simulink model "MPC"  (R2024b)
settings: Solver=ode4  StartTime=0.0  StopTime=tsim  FixedStep=baseRate  RelTol=1e-6  AbsTol=1e-6
values from neighbouring files (symbols this model uses):
  IBLACK = 0.1996    [unpackData.m]
  IRED = 0.1982    [unpackData.m]
  m = m + 5    (= 4)    [unpackData.m]
  M = diag([1/m; 1/m; 1/I])    [unpackData.m]
  mBLACK = 11.3620    (= 11.362)    [unpackData.m]
  mRED = 11.2970    (= 11.297)    [unpackData.m]
  N = 0    [unpackData.m]
  Q = blkdiag(0.0001*eye(2), 0.00001)    [unpackData.m]
  R = diag([6;6;6])    [unpackData.m]
undefined symbols (not defined in the file or in its folder): a1, a2, a3, alpha, alpha_m, alpha_t, alphas, alphas_t, alphat, Am, b, b0, b1, b2, b3, baseRate, Bm, C, c, c1, c1t, c2, c2t, camera_FOV, camera_offset, Cm, d, dataRate, DiscIntNeverNeededParam, Dm, docking_face, docking_offset, drop_states_ARM, drop_states_BLACK, drop_states_BLUE, drop_states_RED, epsilon, epsilont, eta, F_black_X_nominal, F_black_Y_nominal, F_blue_X_nominal, F_blue_Y_nominal, F_max, F_red_X_nominal, F_red_Y_nominal, f_t, F_t, F_thrusters_BLACK, F_thrusters_BLUE, F_thrusters_RED, F_u, f_u, F_v, gamma, Gamma1_el, Gamma1_sh, Gamma1_wr, Gamma2_el, Gamma2_sh ... (+118)
libraries: simulink x33, nvidiaSharedBlocks x13, slpidlib x6, MainLibrary x5, dspsigops x3, dspinverses x3, nvidiaIMUSensorslib x1
(part 2 of 11)

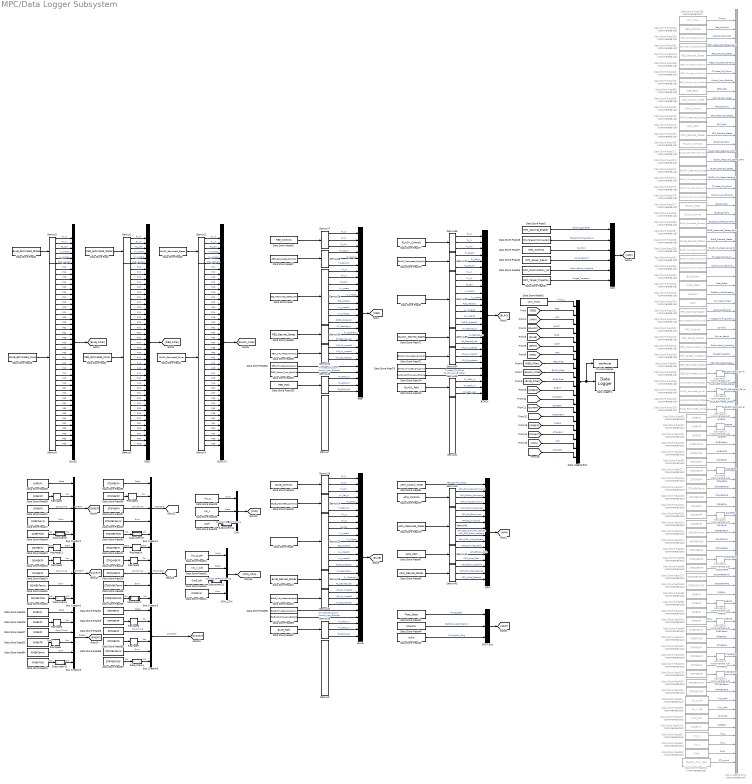
== system MPC/Data Logger Subsystem ==
  ARM : BusCreator  Inputs=16
  BLACK : BusCreator  Inputs=26
  BLACK2 : BusCreator  Inputs=42
  BLUE : BusCreator  Inputs=26
  BLUE2 : BusCreator  Inputs=42
  Bus Creator{1..4} (4 alike) : BusCreator  Inputs=5
  Bus Creator5 : BusCreator  Inputs=6
  Bus Creator6 : BusCreator  Inputs=6
  CNN : BusCreator  Inputs=3
  CNN_ZOH : BusCreator  Inputs=4
  Data Logger1 : MainLibrary/Data Logger  SystemSampleTime=-1  VariantActivationTime=update diagram  AllowFlexibleInterface=on  Latency=0  AutoFrameSizeCalculation=off
      settings: SourceProductName=SPOT Custom Library
  Data Logging Bus : BusCreator  Inputs=18
  Data Logging Bus1 : BusCreator  Commented=on  Inputs=85
  Data Store Read : DataStoreRead  DataStoreName=RED_Estimated_States  IndexOptions=Index vector (dialog)  Indices=1  OutputSizes=1
  Data Store Read1 : DataStoreRead  DataStoreName=MPC_Docking_Enabler  IndexOptions=Index vector (dialog)  Indices=1  OutputSizes=1
  Data Store Read10 : DataStoreRead  DataStoreName=STDQMEKFx  IndexOptions=Index vector (dialog)  Indices=1  OutputSizes=1
  Data Store Read100 : DataStoreRead  Commented=on  DataStoreName=Conf_zoh  IndexOptions=Index vector (dialog)  Indices=1  OutputSizes=1
  Data Store Read101 : DataStoreRead  Commented=on  DataStoreName=CNNError  IndexOptions=Index vector (dialog)  Indices=1  OutputSizes=1
  Data Store Read102 : DataStoreRead  Commented=on  DataStoreName=Float_State  IndexOptions=Index vector (dialog)  Indices=1  OutputSizes=1
  Data Store Read103 : DataStoreRead  Commented=on  DataStoreName=WhoAmI  IndexOptions=Index vector (dialog)  Indices=1  OutputSizes=1
  Data Store Read104 : DataStoreRead  Commented=on  DataStoreName=isSim  IndexOptions=Index vector (dialog)  Indices=1  OutputSizes=1
  Data Store Read105 : DataStoreRead  Commented=on  DataStoreName=RED_Estimated_Covar  IndexOptions=Index vector (dialog)  Indices=1  OutputSizes=1
  Data Store Read108 : DataStoreRead  Commented=on  DataStoreName=QMEKFerror  IndexOptions=Index vector (dialog)  Indices=1  OutputSizes=1
  Data Store Read11 : DataStoreRead  DataStoreName=QMEKFt  IndexOptions=Index vector (dialog)  Indices=1  OutputSizes=1
  Data Store Read114 : DataStoreRead  Commented=on  DataStoreName=DQMEKFerror  IndexOptions=Index vector (dialog)  Indices=1  OutputSizes=1
  Data Store Read115 : DataStoreRead  Commented=on  DataStoreName=DQMEKFNIS  IndexOptions=Index vector (dialog)  Indices=1  OutputSizes=1
  Data Store Read116 : DataStoreRead  Commented=on  DataStoreName=DQMEKFx  IndexOptions=Index vector (dialog)  Indices=1  OutputSizes=1
  Data Store Read117 : DataStoreRead  Commented=on  DataStoreName=STQMEKFP  IndexOptions=Index vector (dialog)  Indices=1  OutputSizes=1
  Data Store Read118 : DataStoreRead  Commented=on  DataStoreName=STQMEKFt  IndexOptions=Index vector (dialog)  Indices=1  OutputSizes=1
  Data Store Read119 : DataStoreRead  Commented=on  DataStoreName=QMEKFNIS  IndexOptions=Index vector (dialog)  Indices=1  OutputSizes=1
  Data Store Read12 : DataStoreRead  DataStoreName=DQMEKFx  IndexOptions=Index vector (dialog)  Indices=1  OutputSizes=1
  Data Store Read120 : DataStoreRead  Commented=on  DataStoreName=BLUE_Estimated_States  IndexOptions=Index vector (dialog)  Indices=1  OutputSizes=1
  Data Store Read122 : DataStoreRead  Commented=on  DataStoreName=MPC_Controls  IndexOptions=Index vector (dialog)  Indices=1  OutputSizes=1
  Data Store Read123 : DataStoreRead  Commented=on  DataStoreName=MPC_Solver_Result  IndexOptions=Index vector (dialog)  Indices=1  OutputSizes=1
  Data Store Read124 : DataStoreRead  Commented=on  DataStoreName=MPC_Target_Holding_Radius  IndexOptions=Index vector (dialog)  Indices=1  OutputSizes=1
  Data Store Read125 : DataStoreRead  Commented=on  DataStoreName=MPC_Optimization_Var  IndexOptions=Index vector (dialog)  Indices=1  OutputSizes=1
  Data Store Read126 : DataStoreRead  Commented=on  DataStoreName=BLUE_Estimated_Covar  IndexOptions=Index vector (dialog)  Indices=1  OutputSizes=1
  Data Store Read127 : DataStoreRead  Commented=on  DataStoreName=STQMEKFerror  IndexOptions=Index vector (dialog)  Indices=1  OutputSizes=1
  Data Store Read128 : DataStoreRead  Commented=on  DataStoreName=STQMEKFNIS  IndexOptions=Index vector (dialog)  Indices=1  OutputSizes=1
  Data Store Read129 : DataStoreRead  Commented=on  DataStoreName=DQMEKFP  IndexOptions=Index vector (dialog)  Indices=1  OutputSizes=1
  Data Store Read13 : DataStoreRead  DataStoreName=DQMEKFP  IndexOptions=Index vector (dialog)  Indices=1  OutputSizes=1
  Data Store Read130 : DataStoreRead  Commented=on  DataStoreName=QMEKFt  IndexOptions=Index vector (dialog)  Indices=1  OutputSizes=1
  Data Store Read131 : DataStoreRead  Commented=on  DataStoreName=DQMEKFt  IndexOptions=Index vector (dialog)  Indices=1  OutputSizes=1
  Data Store Read132 : DataStoreRead  Commented=on  DataStoreName=RMEKFt  IndexOptions=Index vector (dialog)  Indices=1  OutputSizes=1
  Data Store Read133 : DataStoreRead  DataStoreName=RED_Path  IndexOptions=Index vector (dialog)  Indices=1  OutputSizes=1
  Data Store Read134 : DataStoreRead  Commented=on  DataStoreName=RMEKFR  IndexOptions=Index vector (dialog)  Indices=1  OutputSizes=1
  Data Store Read135 : DataStoreRead  Commented=on  DataStoreName=BLACK_Estimated_Covar  IndexOptions=Index vector (dialog)  Indices=1  OutputSizes=1
  Data Store Read136 : DataStoreRead  Commented=on  DataStoreName=BLACK_Estimated_States  IndexOptions=Index vector (dialog)  Indices=1  OutputSizes=1
  Data Store Read137 : DataStoreRead  Commented=on  DataStoreName=STDQMEKFerror  IndexOptions=Index vector (dialog)  Indices=1  OutputSizes=1
  Data Store Read138 : DataStoreRead  Commented=on  DataStoreName=STDQMEKFNIS  IndexOptions=Index vector (dialog)  Indices=1  OutputSizes=1
  Data Store Read139 : DataStoreRead  Commented=on  DataStoreName=RED_Saturated_Controls  IndexOptions=Index vector (dialog)  Indices=1  OutputSizes=1
  Data Store Read14 : DataStoreRead  DataStoreName=DQMEKFt  IndexOptions=Index vector (dialog)  Indices=1  OutputSizes=1
  Data Store Read142 : DataStoreRead  Commented=on  DataStoreName=RMEKFNIS  IndexOptions=Index vector (dialog)  Indices=1  OutputSizes=1
  Data Store Read144 : DataStoreRead  Commented=on  DataStoreName=RED_Controls  IndexOptions=Index vector (dialog)  Indices=1  OutputSizes=1
  Data Store Read145 : DataStoreRead  Commented=on  DataStoreName=RED_Thruster_ON_Count  IndexOptions=Index vector (dialog)  Indices=1  OutputSizes=1
  Data Store Read146 : DataStoreRead  Commented=on  DataStoreName=RED_Control_Law_Enabler  IndexOptions=Index vector (dialog)  Indices=1  OutputSizes=1
  Data Store Read148 : DataStoreRead  Commented=on  DataStoreName=RED_Desired_States  IndexOptions=Index vector (dialog)  Indices=1  OutputSizes=1
  Data Store Read149 : DataStoreRead  Commented=on  DataStoreName=RED_IMU_Measurements  IndexOptions=Index vector (dialog)  Indices=1  OutputSizes=1
  Data Store Read15 : DataStoreRead  DataStoreName=RMEKFx  IndexOptions=Index vector (dialog)  Indices=1  OutputSizes=1
  Data Store Read150 : DataStoreRead  Commented=on  DataStoreName=MPC_Target_Trajectory  IndexOptions=Index vector (dialog)  Indices=1  OutputSizes=1
  Data Store Read151 : DataStoreRead  Commented=on  DataStoreName=MPC_Docking_Enabler  IndexOptions=Index vector (dialog)  Indices=1  OutputSizes=1
  Data Store Read152 : DataStoreRead  Commented=on  DataStoreName=STRMEKFx  IndexOptions=Index vector (dialog)  Indices=1  OutputSizes=1
  Data Store Read153 : DataStoreRead  Commented=on  DataStoreName=RED_Measured_States_RAW  IndexOptions=Index vector (dialog)  Indices=1  OutputSizes=1
  Data Store Read154 : DataStoreRead  Commented=on  DataStoreName=BLACK_CTL_Input  IndexOptions=Index vector (dialog)  Indices=1  OutputSizes=1
  Data Store Read155 : DataStoreRead  Commented=on  DataStoreName=BLUE_Controls  IndexOptions=Index vector (dialog)  Indices=1  OutputSizes=1
  Data Store Read156 : DataStoreRead  Commented=on  DataStoreName=BLUE_Saturated_Controls  IndexOptions=Index vector (dialog)  Indices=1  OutputSizes=1
  Data Store Read157 : DataStoreRead  Commented=on  DataStoreName=BLUE_Measured_States_RAW  IndexOptions=Index vector (dialog)  Indices=1  OutputSizes=1
  Data Store Read158 : DataStoreRead  Commented=on  DataStoreName=BLUE_Desired_States  IndexOptions=Index vector (dialog)  Indices=1  OutputSizes=1
  Data Store Read159 : DataStoreRead  Commented=on  DataStoreName=BLUE_IMU_Measurements  IndexOptions=Index vector (dialog)  Indices=1  OutputSizes=1
  Data Store Read16 : DataStoreRead  DataStoreName=RMEKFP  IndexOptions=Index vector (dialog)  Indices=1  OutputSizes=1
  Data Store Read160 : DataStoreRead  Commented=on  DataStoreName=BLUE_Thruster_ON_Count  IndexOptions=Index vector (dialog)  Indices=1  OutputSizes=1
  Data Store Read161 : DataStoreRead  Commented=on  DataStoreName=BLUE_Control_Law_Enabler  IndexOptions=Index vector (dialog)  Indices=1  OutputSizes=1
  Data Store Read162 : DataStoreRead  Commented=on  DataStoreName=ARM_Measured_States  IndexOptions=Index vector (dialog)  Indices=1  OutputSizes=1
  Data Store Read163 : DataStoreRead  Commented=on  DataStoreName=ARM_Controls  IndexOptions=Index vector (dialog)  Indices=1  OutputSizes=1
  Data Store Read164 : DataStoreRead  Commented=on  DataStoreName=BLUE_Path  IndexOptions=Index vector (dialog)  Indices=1  OutputSizes=1
  Data Store Read165 : DataStoreRead  Commented=on  DataStoreName=BLACK_Controls  IndexOptions=Index vector (dialog)  Indices=1  OutputSizes=1
  Data Store Read166 : DataStoreRead  Commented=on  DataStoreName=ARM_Control_Mode  IndexOptions=Index vector (dialog)  Indices=1  OutputSizes=1
  Data Store Read167 : DataStoreRead  Commented=on  DataStoreName=ARM_Desired_States  IndexOptions=Index vector (dialog)  Indices=1  OutputSizes=1
  Data Store Read168 : DataStoreRead  Commented=on  DataStoreName=STRMEKFP  IndexOptions=Index vector (dialog)  Indices=1  OutputSizes=1
  Data Store Read169 : DataStoreRead  Commented=on  DataStoreName=Univ_Time  IndexOptions=Index vector (dialog)  Indices=1  OutputSizes=1
  Data Store Read17 : DataStoreRead  DataStoreName=RMEKFt  IndexOptions=Index vector (dialog)  Indices=1  OutputSizes=1
  Data Store Read170 : DataStoreRead  Commented=on  DataStoreName=ARM_Path  IndexOptions=Index vector (dialog)  Indices=1  OutputSizes=1
  Data Store Read171 : DataStoreRead  Commented=on  DataStoreName=BLACK_Saturated_Controls  IndexOptions=Index vector (dialog)  Indices=1  OutputSizes=1
  Data Store Read172 : DataStoreRead  Commented=on  DataStoreName=BLACK_Measured_States_RAW  IndexOptions=Index vector (dialog)  Indices=1  OutputSizes=1
  Data Store Read173 : DataStoreRead  Commented=on  DataStoreName=BLACK_Desired_States  IndexOptions=Index vector (dialog)  Indices=1  OutputSizes=1
  Data Store Read174 : DataStoreRead  Commented=on  DataStoreName=BLACK_IMU_Measurements  IndexOptions=Index vector (dialog)  Indices=1  OutputSizes=1
  Data Store Read175 : DataStoreRead  Commented=on  DataStoreName=BLACK_Thruster_ON_Count  IndexOptions=Index vector (dialog)  Indices=1  OutputSizes=1
  Data Store Read176 : DataStoreRead  Commented=on  DataStoreName=BLACK_Control_Law_Enabler  IndexOptions=Index vector (dialog)  Indices=1  OutputSizes=1
  Data Store Read177 : DataStoreRead  Commented=on  DataStoreName=BLACK_Path  IndexOptions=Index vector (dialog)  Indices=1  OutputSizes=1
  Data Store Read178 : DataStoreRead  Commented=on  DataStoreName=STRMEKFt  IndexOptions=Index vector (dialog)  Indices=1  OutputSizes=1
  Data Store Read179 : DataStoreRead  Commented=on  DataStoreName=STRMEKFR  IndexOptions=Index vector (dialog)  Indices=1  OutputSizes=1
  Data Store Read18 : DataStoreRead  DataStoreName=STDQMEKFP  IndexOptions=Index vector (dialog)  Indices=1  OutputSizes=1
  Data Store Read180 : DataStoreRead  Commented=on  DataStoreName=STRMEKFerror  IndexOptions=Index vector (dialog)  Indices=1  OutputSizes=1
  Data Store Read181 : DataStoreRead  Commented=on  DataStoreName=STRMEKFNIS  IndexOptions=Index vector (dialog)  Indices=1  OutputSizes=1
  Data Store Read19 : DataStoreRead  DataStoreName=STDQMEKFt  IndexOptions=Index vector (dialog)  Indices=1  OutputSizes=1
  Data Store Read2 : DataStoreRead  DataStoreName=RED_Estimated_Covar  IndexOptions=Index vector (dialog)  Indices=1  OutputSizes=1
  Data Store Read20 : DataStoreRead  DataStoreName=RMEKFR  IndexOptions=Index vector (dialog)  Indices=1  OutputSizes=1
  Data Store Read21 : DataStoreRead  DataStoreName=RMEKFNIS  IndexOptions=Index vector (dialog)  Indices=1  OutputSizes=1
  Data Store Read22 : DataStoreRead  DataStoreName=STRMEKFx  IndexOptions=Index vector (dialog)  Indices=1  OutputSizes=1
  Data Store Read23 : DataStoreRead  DataStoreName=STRMEKFP  IndexOptions=Index vector (dialog)  Indices=1  OutputSizes=1
  Data Store Read24 : DataStoreRead  DataStoreName=BLUE_Desired_States  IndexOptions=Index vector (dialog)  Indices=1  OutputSizes=1
  Data Store Read25 : DataStoreRead  DataStoreName=BLUE_IMU_Measurements  IndexOptions=Index vector (dialog)  Indices=1  OutputSizes=1
  Data Store Read26 : DataStoreRead  DataStoreName=BLUE_Saturated_Controls  IndexOptions=Index vector (dialog)  Indices=1  OutputSizes=1
  Data Store Read27 : DataStoreRead  DataStoreName=MPC_Controls  IndexOptions=Index vector (dialog)  Indices=1  OutputSizes=1
  Data Store Read28 : DataStoreRead  DataStoreName=STRMEKFt  IndexOptions=Index vector (dialog)  Indices=1  OutputSizes=1
  Data Store Read29 : DataStoreRead  DataStoreName=Vis_q  IndexOptions=Index vector (dialog)  Indices=1  OutputSizes=1
  Data Store Read3 : DataStoreRead  DataStoreName=BLACK_Estimated_States  IndexOptions=Index vector (dialog)  Indices=1  OutputSizes=1
  Data Store Read30 : DataStoreRead  DataStoreName=Vis_x  IndexOptions=Index vector (dialog)  Indices=1  OutputSizes=1
  Data Store Read31 : DataStoreRead  DataStoreName=Vis_q_zoh  IndexOptions=Index vector (dialog)  Indices=1  OutputSizes=1
  Data Store Read32 : DataStoreRead  DataStoreName=Vis_x_zoh  IndexOptions=Index vector (dialog)  Indices=1  OutputSizes=1
  Data Store Read33 : DataStoreRead  DataStoreName=Conf  IndexOptions=Index vector (dialog)  Indices=1  OutputSizes=1
  Data Store Read34 : DataStoreRead  DataStoreName=Conf_zoh  IndexOptions=Index vector (dialog)  Indices=1  OutputSizes=1
  Data Store Read35 : DataStoreRead  DataStoreName=STQMEKFx  IndexOptions=Index vector (dialog)  Indices=1  OutputSizes=1
  Data Store Read36 : DataStoreRead  DataStoreName=STQMEKFP  IndexOptions=Index vector (dialog)  Indices=1  OutputSizes=1
  Data Store Read37 : DataStoreRead  DataStoreName=STQMEKFt  IndexOptions=Index vector (dialog)  Indices=1  OutputSizes=1
  Data Store Read38 : DataStoreRead  DataStoreName=QMEKFx  IndexOptions=Index vector (dialog)  Indices=1  OutputSizes=1
  Data Store Read39 : DataStoreRead  DataStoreName=QMEKFP  IndexOptions=Index vector (dialog)  Indices=1  OutputSizes=1
  Data Store Read4 : DataStoreRead  DataStoreName=BLACK_Estimated_Covar  IndexOptions=Index vector (dialog)  Indices=1  OutputSizes=1
  Data Store Read40 : DataStoreRead  DataStoreName=MPC_Solver_Result  IndexOptions=Index vector (dialog)  Indices=1  OutputSizes=1
  Data Store Read41 : DataStoreRead  DataStoreName=CNNError  IndexOptions=Index vector (dialog)  Indices=1  OutputSizes=1
  Data Store Read42 : DataStoreRead  DataStoreName=Float_State  IndexOptions=Index vector (dialog)  Indices=1  OutputSizes=1
  Data Store Read43 : DataStoreRead  DataStoreName=BLUE_Controls  IndexOptions=Index vector (dialog)  Indices=1  OutputSizes=1
  Data Store Read44 : DataStoreRead  DataStoreName=WhoAmI  IndexOptions=Index vector (dialog)  Indices=1  OutputSizes=1
  Data Store Read45 : DataStoreRead  DataStoreName=isSim  IndexOptions=Index vector (dialog)  Indices=1  OutputSizes=1
  Data Store Read46 : DataStoreRead  DataStoreName=MPC_Target_Holding_Radius  IndexOptions=Index vector (dialog)  Indices=1  OutputSizes=1
  Data Store Read47 : DataStoreRead  DataStoreName=QMEKFerror  IndexOptions=Index vector (dialog)  Indices=1  OutputSizes=1
  Data Store Read48 : DataStoreRead  DataStoreName=QMEKFNIS  IndexOptions=Index vector (dialog)  Indices=1  OutputSizes=1
  Data Store Read49 : DataStoreRead  DataStoreName=STQMEKFerror  IndexOptions=Index vector (dialog)  Indices=1  OutputSizes=1
  Data Store Read5 : DataStoreRead  DataStoreName=BLUE_Estimated_States  IndexOptions=Index vector (dialog)  Indices=1  OutputSizes=1
  Data Store Read50 : DataStoreRead  DataStoreName=STQMEKFNIS  IndexOptions=Index vector (dialog)  Indices=1  OutputSizes=1
  Data Store Read51 : DataStoreRead  DataStoreName=DQMEKFerror  IndexOptions=Index vector (dialog)  Indices=1  OutputSizes=1
  Data Store Read52 : DataStoreRead  DataStoreName=DQMEKFNIS  IndexOptions=Index vector (dialog)  Indices=1  OutputSizes=1
  Data Store Read53 : DataStoreRead  DataStoreName=MPC_Optimization_Var  IndexOptions=Index vector (dialog)  Indices=1  OutputSizes=1
  Data Store Read54 : DataStoreRead  DataStoreName=MPC_Target_Trajectory  IndexOptions=Index vector (dialog)  Indices=1  OutputSizes=1
  Data Store Read55 : DataStoreRead  DataStoreName=STDQMEKFerror  IndexOptions=Index vector (dialog)  Indices=1  OutputSizes=1
  Data Store Read56 : DataStoreRead  DataStoreName=STDQMEKFNIS  IndexOptions=Index vector (dialog)  Indices=1  OutputSizes=1
  Data Store Read57 : DataStoreRead  DataStoreName=RED_Saturated_Controls  IndexOptions=Index vector (dialog)  Indices=1  OutputSizes=1
  Data Store Read58 : DataStoreRead  DataStoreName=STRMEKFR  IndexOptions=Index vector (dialog)  Indices=1  OutputSizes=1
  Data Store Read59 : DataStoreRead  DataStoreName=STRMEKFerror  IndexOptions=Index vector (dialog)  Indices=1  OutputSizes=1
  Data Store Read6 : DataStoreRead  DataStoreName=BLUE_Estimated_Covar  IndexOptions=Index vector (dialog)  Indices=1  OutputSizes=1
  Data Store Read60 : DataStoreRead  DataStoreName=STRMEKFNIS  IndexOptions=Index vector (dialog)  Indices=1  OutputSizes=1
  Data Store Read61 : DataStoreRead  DataStoreName=RED_Controls  IndexOptions=Index vector (dialog)  Indices=1  OutputSizes=1
  Data Store Read62 : DataStoreRead  DataStoreName=RED_Thruster_ON_Count  IndexOptions=Index vector (dialog)  Indices=1  OutputSizes=1
  Data Store Read63 : DataStoreRead  DataStoreName=RED_Control_Law_Enabler  IndexOptions=Index vector (dialog)  Indices=1  OutputSizes=1
  Data Store Read64 : DataStoreRead  DataStoreName=RMEKFerror  IndexOptions=Index vector (dialog)  Indices=1  OutputSizes=1
  Data Store Read65 : DataStoreRead  DataStoreName=RED_Desired_States  IndexOptions=Index vector (dialog)  Indices=1  OutputSizes=1
  Data Store Read66 : DataStoreRead  DataStoreName=RED_IMU_Measurements  IndexOptions=Index vector (dialog)  Indices=1  OutputSizes=1
  Data Store Read67 : DataStoreRead  DataStoreName=BLUE_Path  IndexOptions=Index vector (dialog)  Indices=1  OutputSizes=1
  Data Store Read68 : DataStoreRead  DataStoreName=BLUE_Thruster_ON_Count  IndexOptions=Index vector (dialog)  Indices=1  OutputSizes=1
  Data Store Read69 : DataStoreRead  DataStoreName=BLUE_Control_Law_Enabler  IndexOptions=Index vector (dialog)  Indices=1  OutputSizes=1
  Data Store Read7 : DataStoreRead  DataStoreName=RED_Measured_States_RAW  IndexOptions=Index vector (dialog)  Indices=1  OutputSizes=1
  Data Store Read71 : DataStoreRead  DataStoreName=BLACK_Desired_States  IndexOptions=Index vector (dialog)  Indices=1  OutputSizes=1
  Data Store Read72 : DataStoreRead  DataStoreName=BLACK_IMU_Measurements  IndexOptions=Index vector (dialog)  Indices=1  OutputSizes=1
  Data Store Read73 : DataStoreRead  DataStoreName=BLACK_Thruster_ON_Count  IndexOptions=Index vector (dialog)  Indices=1  OutputSizes=1
  Data Store Read74 : DataStoreRead  DataStoreName=BLACK_Control_Law_Enabler  IndexOptions=Index vector (dialog)  Indices=1  OutputSizes=1
  Data Store Read75 : DataStoreRead  DataStoreName=BLACK_Saturated_Controls  IndexOptions=Index vector (dialog)  Indices=1  OutputSizes=1
  Data Store Read76 : DataStoreRead  DataStoreName=BLACK_Path  IndexOptions=Index vector (dialog)  Indices=1  OutputSizes=1
  Data Store Read77 : DataStoreRead  DataStoreName=BLACK_Controls  IndexOptions=Index vector (dialog)  Indices=1  OutputSizes=1
  Data Store Read78 : DataStoreRead  DataStoreName=ARM_Measured_States  IndexOptions=Index vector (dialog)  Indices=1  OutputSizes=1
  Data Store Read79 : DataStoreRead  DataStoreName=ARM_Controls  IndexOptions=Index vector (dialog)  Indices=1  OutputSizes=1
  Data Store Read8 : DataStoreRead  DataStoreName=BLACK_Measured_States_RAW  IndexOptions=Index vector (dialog)  Indices=1  OutputSizes=1
  Data Store Read80 : DataStoreRead  DataStoreName=ARM_Desired_States  IndexOptions=Index vector (dialog)  Indices=1  OutputSizes=1
  Data Store Read81 : DataStoreRead  DataStoreName=ARM_Control_Mode  IndexOptions=Index vector (dialog)  Indices=1  OutputSizes=1
  Data Store Read82 : DataStoreRead  Commented=on  DataStoreName=QMEKFx  IndexOptions=Index vector (dialog)  Indices=1  OutputSizes=1
  Data Store Read83 : DataStoreRead  Commented=on  DataStoreName=RED_Estimated_States  IndexOptions=Index vector (dialog)  Indices=1  OutputSizes=1
  Data Store Read84 : DataStoreRead  Commented=on  DataStoreName=STDQMEKFx  IndexOptions=Index vector (dialog)  Indices=1  OutputSizes=1
  Data Store Read85 : DataStoreRead  Commented=on  DataStoreName=STQMEKFx  IndexOptions=Index vector (dialog)  Indices=1  OutputSizes=1
  Data Store Read86 : DataStoreRead  Commented=on  DataStoreName=RMEKFerror  IndexOptions=Index vector (dialog)  Indices=1  OutputSizes=1
  Data Store Read87 : DataStoreRead  DataStoreName=ARM_Path  IndexOptions=Index vector (dialog)  Indices=1  OutputSizes=1
  Data Store Read88 : DataStoreRead  Commented=on  DataStoreName=RMEKFx  IndexOptions=Index vector (dialog)  Indices=1  OutputSizes=1
  Data Store Read89 : DataStoreRead  Commented=on  DataStoreName=RED_Path  IndexOptions=Index vector (dialog)  Indices=1  OutputSizes=1
  Data Store Read9 : DataStoreRead  DataStoreName=BLUE_Measured_States_RAW  IndexOptions=Index vector (dialog)  Indices=1  OutputSizes=1
  Data Store Read90 : DataStoreRead  Commented=on  DataStoreName=RMEKFP  IndexOptions=Index vector (dialog)  Indices=1  OutputSizes=1
  Data Store Read91 : DataStoreRead  DataStoreName=Univ_Time  IndexOptions=Index vector (dialog)  Indices=1  OutputSizes=1
  Data Store Read92 : DataStoreRead  Commented=on  DataStoreName=Vis_q  IndexOptions=Index vector (dialog)  Indices=1  OutputSizes=1
  Data Store Read93 : DataStoreRead  Commented=on  DataStoreName=Vis_x  IndexOptions=Index vector (dialog)  Indices=1  OutputSizes=1
  Data Store Read94 : DataStoreRead  Commented=on  DataStoreName=Vis_q_zoh  IndexOptions=Index vector (dialog)  Indices=1  OutputSizes=1
  Data Store Read95 : DataStoreRead  Commented=on  DataStoreName=STDQMEKFP  IndexOptions=Index vector (dialog)  Indices=1  OutputSizes=1
  Data Store Read96 : DataStoreRead  Commented=on  DataStoreName=STDQMEKFt  IndexOptions=Index vector (dialog)  Indices=1  OutputSizes=1
  Data Store Read97 : DataStoreRead  Commented=on  DataStoreName=QMEKFP  IndexOptions=Index vector (dialog)  Indices=1  OutputSizes=1
  Data Store Read98 : DataStoreRead  Commented=on  DataStoreName=Vis_x_zoh  IndexOptions=Index vector (dialog)  Indices=1  OutputSizes=1
  Data Store Read99 : DataStoreRead  Commented=on  DataStoreName=Conf  IndexOptions=Index vector (dialog)  Indices=1  OutputSizes=1
  Demux{1,3,5,41} (4 alike) : Demux  Outputs=6
  Demux2 : Demux  Outputs=36
  Demux{22..24,26..28,30..31,33..37,39..40,42..43,48} (18 alike) : Demux  Outputs=3
  Demux{7..9,25,29,38} (6 alike) : Demux  Outputs=9
  Demux4 : Demux  Outputs=36
  Demux6 : Demux  Outputs=36
  MPC : BusCreator  Inputs=6
  RED : BusCreator  Inputs=26
  RED2 : BusCreator  Inputs=42
  Reshape{1..8,13..14} (10 alike) : Reshape
  Reshape{9..12,17..23} (11 alike) : Reshape  Commented=on
  SPOT Bus : BusCreator  Inputs=3
  Subsystem1 : Subsystem
  Subsystem11 : Subsystem
  Subsystem13 : Subsystem
  Subsystem14 : Subsystem
  Subsystem17 : Subsystem
  Subsystem3 : Subsystem
  Subsystem4 : Subsystem
  Subsystem8 : Subsystem
  To Workspace1 : ToWorkspace  VariableName=dataPacket  SaveFormat=Timeseries  SampleTime=-1
      settings: Save2DSignal=2-D array (concatenate along first dimension)
  wires:
  Data Store Read24/1 -> Demux26/1
  Data Store Read43/1 -> Demux23/1
  Data Store Read26/1 -> Demux24/1
  Demux23/1 -> BLUE/1  "Fx_N"
  Demux23/2 -> BLUE/2  "Fy_N"
  Demux23/3 -> BLUE/3  "Tz_Nm"
  Demux24/1 -> BLUE/4  "Fx_Sat_N"
  Demux24/2 -> BLUE/5  "Fy_Sat_N"
  Demux24/3 -> BLUE/6  "Tz_Sat_Nm"
  Demux25/1 -> BLUE/7  "Px_m"
  Demux25/2 -> BLUE/8  "Py_m"
  Demux25/3 -> BLUE/9  "Rz_rad"
  Demux25/4 -> BLUE/10  "Vx_mpers"
  Demux25/5 -> BLUE/11  "Vy_mpers"
  Demux25/6 -> BLUE/12  "RzD_radpers"
  Demux25/7 -> BLUE/13  "Ax_mpers2"
  Demux25/8 -> BLUE/14  "Ay_mpers2"
  Demux25/9 -> BLUE/15  "RzDD_radpers2"
  Demux26/1 -> BLUE/16  "Px_Desired_m"
  Demux26/2 -> BLUE/17  "Py_Desired_m"
  Demux26/3 -> BLUE/18  "Rz_Desired_rad"
  Demux22/1 -> BLUE/19  "IMU_Ax_mpers2"
  Demux22/2 -> BLUE/20  "IMU_Ay_mpers2"
  Demux22/3 -> BLUE/21  "IMU_Gz_radpers"
  Data Store Read25/1 -> Demux22/1
  Data Store Read57/1 -> Demux28/1
  Data Store Read66/1 -> Demux31/1
  Data Store Read65/1 -> Demux30/1
  Data Store Read67/1 -> Demux33/1
  Data Store Read68/1 -> BLUE/22  "Thruster_ON_Count"
  Data Store Read69/1 -> BLUE/23  "Control_Law_Enabler"
  Data Store Read62/1 -> RED/22  "Thruster_ON_Count"
  Data Store Read63/1 -> RED/23  "Control_Law_Enabler"
  Demux29/9 -> RED/15  "RzDD_radpers2"
  Demux31/3 -> RED/21  "IMU_Gz_radpers"
  Demux28/3 -> RED/6  "Tz_Sat_Nm"
  Demux30/1 -> RED/16  "Px_Desired_m"
  Demux30/3 -> RED/18  "Rz_Desired_rad"
  Demux31/2 -> RED/20  "IMU_Ay_mpers2"
  Demux30/2 -> RED/17  "Py_Desired_m"
  Demux29/5 -> RED/11  "Vy_mpers"
  Demux29/4 -> RED/10  "Vx_mpers"
  Demux29/7 -> RED/13  "Ax_mpers2"
  Demux28/2 -> RED/5  "Fy_Sat_N"
  Demux29/6 -> RED/12  "RzD_radpers"
  Demux29/8 -> RED/14  "Ay_mpers2"
  Demux31/1 -> RED/19  "IMU_Ax_mpers2"
  Demux29/1 -> RED/7  "Px_m"
  Demux27/2 -> RED/2  "Fy_N"
  Demux29/2 -> RED/8  "Py_m"
  Demux27/1 -> RED/1  "Fx_N"
  Demux27/3 -> RED/3  "Tz_Nm"
  Demux28/1 -> RED/4  "Fx_Sat_N"
  Demux29/3 -> RED/9  "Rz_rad"
  Data Store Read61/1 -> Demux27/1
  Data Store Read72/1 -> Demux34/1
  Data Store Read75/1 -> Demux37/1
  Data Store Read76/1 -> Demux35/1
  Data Store Read77/1 -> Demux36/1
  Data Store Read71/1 -> Demux39/1
  Data Store Read73/1 -> BLACK/22  "Thruster_ON_Count"
  Data Store Read74/1 -> BLACK/23  "Control_Law_Enabler"
  Demux35/1 -> BLACK/24  "Px_Path_m"
  Demux35/2 -> BLACK/25  "Py_Path_m"
  Demux35/3 -> BLACK/26  "Rz_Path_rad"
  Demux34/3 -> BLACK/21  "IMU_Gz_radpers"
  Demux34/2 -> BLACK/20  "IMU_Ay_mpers2"
  Demux34/1 -> BLACK/19  "IMU_Ax_mpers2"
  Demux39/3 -> BLACK/18  "Rz_Desired_rad"
  Demux39/2 -> BLACK/17  "Py_Desired_m"
  Demux39/1 -> BLACK/16  "Px_Desired_m"
  Demux38/9 -> BLACK/15  "RzDD_radpers2"
  Demux38/8 -> BLACK/14  "Ay_mpers2"
  Demux38/7 -> BLACK/13  "Ax_mpers2"
  Demux38/6 -> BLACK/12  "RzD_radpers"
  Demux38/5 -> BLACK/11  "Vy_mpers"
  Demux38/4 -> BLACK/10  "Vx_mpers"
  Demux38/3 -> BLACK/9  "Rz_rad"
  Demux38/2 -> BLACK/8  "Py_m"
  Demux38/1 -> BLACK/7  "Px_m"
  Demux37/3 -> BLACK/6  "Tz_Sat_Nm"
  Demux37/2 -> BLACK/5  "Fy_Sat_N"
  Demux37/1 -> BLACK/4  "Fx_Sat_N"
  Demux36/3 -> BLACK/3  "Tz_Nm"
  Demux36/2 -> BLACK/2  "Fy_N"
  Demux36/1 -> BLACK/1  "Fx_N"
  Data Store Read87/1 -> Demux42/1
  Data Store Read79/1 -> Demux40/1
  Data Store Read78/1 -> Demux41/1
  Data Store Read80/1 -> Demux43/1
  Data Store Read81/1 -> ARM/1  "ARM_Control_Mode"
  Demux40/1 -> ARM/2  "ARM_Shoulder_Command"
  Demux40/2 -> ARM/3  "ARM_Elbow_Command"
  Demux40/3 -> ARM/4  "ARM_Wrist_Command"
  Demux41/1 -> ARM/5  "ARM_Rz_Shoulder_rad"
  Demux41/2 -> ARM/6  "ARM_Rz_Elbow_rad"
  Demux41/3 -> ARM/7  "ARM_Rz_Wrist_rad"
  Demux41/4 -> ARM/8  "ARM_RzD_Shoulder_radpers"
  Demux41/5 -> ARM/9  "ARM_RzD_Elbow_radpers"
  Demux41/6 -> ARM/10  "ARM_RzD_Wrist_radpers"
  Demux42/1 -> ARM/11  "ARM_Shoulder_Path"
  Demux42/2 -> ARM/12  "ARM_Elbow_Path"
  Demux42/3 -> ARM/13  "ARM_Wrist_Path"
  Demux43/1 -> ARM/14  "ARM_Elbow_Desired"
  Demux43/2 -> ARM/15  "ARM_Shoulder_Desired"
  Demux43/3 -> ARM/16  "ARM_Wrist_Desired"
  RED/1 -> [RED]
  ARM/1 -> [ARM]
  BLACK/1 -> [BLACK]
  BLUE/1 -> [BLUE]
  Demux48/1 -> RED/24  "Px_Path_m"
  Demux48/2 -> RED/25  "Py_Path_m"
  Demux48/3 -> RED/26  "Rz_Path_rad"
  Data Store Read133/1 -> Demux48/1
  Data Store Read42/1 -> SPOT Bus/1  "Float_State"
  SPOT Bus/1 -> [SPOT]
  Data Store Read45/1 -> SPOT Bus/3  "Simulation_Flag"
  Data Store Read44/1 -> SPOT Bus/2  "Platform_Identification"
  [MPC] -> Data Logging Bus/7  "MPC"
  [RED] -> Data Logging Bus/2  "RED"
  [SPOT] -> Data Logging Bus/6  "SPOT"
  [ARM] -> Data Logging Bus/3  "ARM"
  [BLUE] -> Data Logging Bus/5  "BLUE"
  [BLACK] -> Data Logging Bus/4  "BLACK"
  Data Store Read91/1 -> Data Logging Bus/1  "Time_s"
  MPC/1 -> [MPC]
  Data Store Read1/1 -> MPC/1  "Docking_Enabler"
  Data Store Read54/1 -> MPC/6  "Target_Trajectory"
  Data Store Read53/1 -> MPC/5  "Optimization_Variable"
  Data Store Read40/1 -> MPC/4  "Solver_Result"
  Data Store Read46/1 -> MPC/2  "Target_Holding_Radius"
  Data Store Read27/1 -> MPC/3  "Controls"
  Data Store Read/1 -> Demux1/1
  Data Store Read2/1 -> Demux2/1
  Demux1/6 -> RED2/6  "RzD_radpers"
  Demux1/5 -> RED2/5  "Vy_mpers"
  Demux1/4 -> RED2/4  "Vx_mpers"
  Demux1/3 -> RED2/3  "Rz_rad"
  Demux1/2 -> RED2/2  "Py_m"
  Demux1/1 -> RED2/1  "Px_m"
  Demux2/1 -> RED2/7  "P11"
  Demux2/2 -> RED2/8  "P12"
  Demux2/3 -> RED2/9  "P13"
  Demux2/4 -> RED2/10  "P14"
  Demux2/5 -> RED2/11  "P15"
  Demux2/6 -> RED2/12  "P16"
  Demux2/7 -> RED2/13  "P21"
  Demux2/8 -> RED2/14  "P22"
  Demux2/9 -> RED2/15  "P23"
  Demux2/10 -> RED2/16  "P24"
  Demux2/11 -> RED2/17  "P25"
  Demux2/12 -> RED2/18  "P26"
  Demux2/13 -> RED2/19  "P31"
  Demux2/14 -> RED2/20  "P32"
  Demux2/15 -> RED2/21  "P33"
  Demux2/16 -> RED2/22  "P34"
  Demux2/17 -> RED2/23  "P35"
  Demux2/18 -> RED2/24  "P36"
  Demux2/19 -> RED2/25  "P41"
  Demux2/20 -> RED2/26  "P42"
  Demux2/21 -> RED2/27  "P43"
  Demux2/22 -> RED2/28  "P44"
  Demux2/23 -> RED2/29  "P45"
  Demux2/24 -> RED2/30  "P46"
  Demux2/25 -> RED2/31  "P51"
  Demux2/26 -> RED2/32  "P52"
  Demux2/27 -> RED2/33  "P53"
  Demux2/28 -> RED2/34  "P54"
  Demux2/29 -> RED2/35  "P55"
  Demux2/30 -> RED2/36  "P56"
  Demux2/31 -> RED2/37  "P61"
  Demux2/32 -> RED2/38  "P62"
  Demux2/33 -> RED2/39  "P63"
  Demux2/34 -> RED2/40  "P64"
  Demux2/35 -> RED2/41  "P65"
  Demux2/36 -> RED2/42  "P66"
  RED2/1 -> [RED_Filter]
  Demux4/13 -> BLACK2/19  "P31"
  Demux4/27 -> BLACK2/33  "P53"
  Demux4/18 -> BLACK2/24  "P36"
  Demux4/26 -> BLACK2/32  "P52"
  Demux3/6 -> BLACK2/6  "RzD_radpers"
  Demux3/5 -> BLACK2/5  "Vy_mpers"
  Demux4/2 -> BLACK2/8  "P12"
  Demux4/14 -> BLACK2/20  "P32"
  Demux4/24 -> BLACK2/30  "P46"
  Demux4/16 -> BLACK2/22  "P34"
  Demux3/2 -> BLACK2/2  "Py_m"
  Demux4/29 -> BLACK2/35  "P55"
  Demux4/31 -> BLACK2/37  "P61"
  Demux4/10 -> BLACK2/16  "P24"
  Demux3/4 -> BLACK2/4  "Vx_mpers"
  Demux4/9 -> BLACK2/15  "P23"
  Demux3/3 -> BLACK2/3  "Rz_rad"
  Demux4/12 -> BLACK2/18  "P26"
  Demux4/22 -> BLACK2/28  "P44"
  Data Store Read3/1 -> Demux3/1
  Demux4/23 -> BLACK2/29  "P45"
  Demux4/3 -> BLACK2/9  "P13"
  Demux4/21 -> BLACK2/27  "P43"
  Demux4/30 -> BLACK2/36  "P56"
  Demux4/5 -> BLACK2/11  "P15"
  Demux4/17 -> BLACK2/23  "P35"
  Demux4/20 -> BLACK2/26  "P42"
  Demux4/6 -> BLACK2/12  "P16"
  Demux4/19 -> BLACK2/25  "P41"
  Data Store Read4/1 -> Demux4/1
  Demux4/4 -> BLACK2/10  "P14"
  Demux4/7 -> BLACK2/13  "P21"
  BLACK2/1 -> [BLACK_Filter]
  Demux4/25 -> BLACK2/31  "P51"
  Demux4/28 -> BLACK2/34  "P54"
  Demux4/8 -> BLACK2/14  "P22"
  Demux4/15 -> BLACK2/21  "P33"
  Demux4/11 -> BLACK2/17  "P25"
  Demux3/1 -> BLACK2/1  "Px_m"
  Demux4/1 -> BLACK2/7  "P11"
  Demux5/1 -> BLUE2/1  "Px_m"
  Demux6/25 -> BLUE2/31  "P51"
  BLUE2/1 -> [BLUE_Filter]
  Data Store Read6/1 -> Demux6/1
  Demux6/4 -> BLUE2/10  "P14"
  Demux6/19 -> BLUE2/25  "P41"
  Demux6/28 -> BLUE2/34  "P54"
  Demux6/30 -> BLUE2/36  "P56"
  Demux6/6 -> BLUE2/12  "P16"
  Demux6/21 -> BLUE2/27  "P43"
  Demux6/5 -> BLUE2/11  "P15"
  Demux6/22 -> BLUE2/28  "P44"
  Demux5/3 -> BLUE2/3  "Rz_rad"
  Demux6/12 -> BLUE2/18  "P26"
  Demux6/8 -> BLUE2/14  "P22"
  Demux5/2 -> BLUE2/2  "Py_m"
  Demux6/1 -> BLUE2/7  "P11"
  Demux6/16 -> BLUE2/22  "P34"
  Demux6/31 -> BLUE2/37  "P61"
  Demux6/10 -> BLUE2/16  "P24"
  Demux6/3 -> BLUE2/9  "P13"
  Demux6/9 -> BLUE2/15  "P23"
  Demux5/4 -> BLUE2/4  "Vx_mpers"
  Demux5/6 -> BLUE2/6  "RzD_radpers"
  Demux6/20 -> BLUE2/26  "P42"
  Demux6/24 -> BLUE2/30  "P46"
  Demux6/7 -> BLUE2/13  "P21"
  Demux6/11 -> BLUE2/17  "P25"
  Demux6/18 -> BLUE2/24  "P36"
  Demux6/29 -> BLUE2/35  "P55"
  Demux6/27 -> BLUE2/33  "P53"
  Demux6/23 -> BLUE2/29  "P45"
  Demux6/13 -> BLUE2/19  "P31"
  Demux6/15 -> BLUE2/21  "P33"
  Demux6/26 -> BLUE2/32  "P52"
  Demux6/2 -> BLUE2/8  "P12"
  Demux5/5 -> BLUE2/5  "Vy_mpers"
  Data Store Read5/1 -> Demux5/1
  Demux6/17 -> BLUE2/23  "P35"
  Demux6/14 -> BLUE2/20  "P32"
  Demux4/32 -> BLACK2/38  "P62"
  Demux4/33 -> BLACK2/39  "P63"
  Demux4/34 -> BLACK2/40  "P64"
  Demux4/35 -> BLACK2/41  "P65"
  Demux4/36 -> BLACK2/42  "P66"
  Demux6/32 -> BLUE2/38  "P62"
  Demux6/33 -> BLUE2/39  "P63"
  Demux6/34 -> BLUE2/40  "P64"
  Demux6/35 -> BLUE2/41  "P65"
  Demux6/36 -> BLUE2/42  "P66"
  [RED_Filter] -> Data Logging Bus/8  "RED_Filter"
  [BLACK_Filter] -> Data Logging Bus/9  "BLACK_Filter"
  [BLUE_Filter] -> Data Logging Bus/10  "BLUE_Filter"
  Demux33/1 -> BLUE/24  "Px_Path_m"
  Demux33/2 -> BLUE/25  "Py_Path_m"
  Demux33/3 -> BLUE/26  "Rz_Path_rad"
  Data Store Read8/1 -> Demux38/1
  Data Store Read7/1 -> Demux29/1
  Data Store Read9/1 -> Demux25/1
  Bus Creator3/1 -> [STDQMEKF]  "STDQMEKF"
  Bus Creator4/1 -> [STQMEKF]  "STQMEKF"
  Data Store Read39/1 -> Reshape1/1
  Reshape1/1 -> Bus Creator1/2  "Cov"
  CNN/1 -> [CNN]
  Bus Creator1/1 -> [QMEKF]  "QMEKF"
  Bus Creator2/1 -> [DQMEKF]  "DQMEKF"
  Data Store Read33/1 -> Subsystem14/1(In1)  "Confidence"
  Bus Creator6/1 -> [STRMEKF]  "STRMEKF"
  Bus Creator5/1 -> [RMEKF]  "RMEKF"
  Data Store Read11/1 -> Bus Creator1/3  "CompTime"
  Data Store Read38/1 -> Bus Creator1/1  "State"
  [QMEKF] -> Data Logging Bus/11  "QMEKF"
  [STQMEKF] -> Data Logging Bus/12  "STQMEKF"
  [DQMEKF] -> Data Logging Bus/13  "DQMEKF"
  [STDQMEKF] -> Data Logging Bus/14  "STDQMEKF"
  [RMEKF] -> Data Logging Bus/15  "RMEKF"
  [STRMEKF] -> Data Logging Bus/16  "STRMEKF"
  [CNN] -> Data Logging Bus/17  "CNN"
  Data Store Read32/1 -> CNN_ZOH/2  "State"
  CNN_ZOH/1 -> [CNN_ZOH]
  Data Store Read31/1 -> CNN_ZOH/1  "Quat"
  Data Store Read34/1 -> Subsystem13/1(In1)  "Confidence"
  [CNN_ZOH] -> Data Logging Bus/18  "CNN_ZOH"
  Data Store Read41/1 -> CNN_ZOH/4  "Error"
  Data Store Read47/1 -> Bus Creator1/4  "Error"
  Data Store Read48/1 -> Subsystem8/1(In1)  "NIS"
  Data Store Read35/1 -> Bus Creator4/1  "State"
  Data Store Read36/1 -> Reshape4/1
  Data Store Read37/1 -> Bus Creator4/3  "CompTime"
  Data Store Read49/1 -> Bus Creator4/4  "Error"
  Data Store Read50/1 -> Subsystem17/1(In1)  "NIS"
  Reshape4/1 -> Bus Creator4/2  "Cov"
  Reshape2/1 -> Bus Creator2/2  "Cov"
  Data Store Read52/1 -> Subsystem3/1(In1)  "NIS"
  Data Store Read12/1 -> Reshape13/1  "State"
  Data Store Read14/1 -> Bus Creator2/3  "CompTime"
  Data Store Read51/1 -> Bus Creator2/4  "Error"
  Data Store Read13/1 -> Reshape2/1
  Reshape3/1 -> Bus Creator3/2  "Cov"
  Data Store Read56/1 -> Subsystem1/1(In1)  "NIS"
  Data Store Read10/1 -> Reshape14/1  "State"
  Data Store Read19/1 -> Bus Creator3/3  "CompTime"
  Data Store Read55/1 -> Bus Creator3/4  "Error"
  Data Store Read18/1 -> Reshape3/1
  Reshape5/1 -> Bus Creator5/2  "Cov"
  Data Store Read21/1 -> Subsystem11/1(In1)  "NIS"
  Data Store Read15/1 -> Bus Creator5/1  "State"
  Data Store Read17/1 -> Bus Creator5/3  "CompTime"
  Data Store Read64/1 -> Bus Creator5/5  "Error"
  Reshape6/1 -> Bus Creator6/2  "Cov"
  Data Store Read60/1 -> Subsystem4/1(In1)  "NIS"
  Data Store Read22/1 -> Bus Creator6/1  "State"
  Data Store Read28/1 -> Bus Creator6/3  "CompTime"
  Data Store Read59/1 -> Bus Creator6/5  "Error"
  Data Store Read16/1 -> Reshape5/1
  Data Store Read23/1 -> Reshape6/1
  Data Store Read58/1 -> Reshape7/1
  Reshape7/1 -> Bus Creator6/4  "Rot"
  Data Store Read20/1 -> Reshape8/1  "Error"
  Reshape8/1 -> Bus Creator5/4  "Rot"
  Data Store Read154/1 -> Data Logging Bus1/85  "CTL_Input"
  Data Store Read169/1 -> Data Logging Bus1/1  "Time_s"
  Data Store Read144/1 -> Data Logging Bus1/2  "Red_Controls"
  Data Store Read139/1 -> Data Logging Bus1/3  "Red_Controls_Sat"
  Data Store Read153/1 -> Data Logging Bus1/4  "RED_Measured_States_RAW"
  Data Store Read148/1 -> Data Logging Bus1/5  "RED_Desired_States"
  Data Store Read149/1 -> Data Logging Bus1/6  "RED_IMU_Measurements"
  Data Store Read145/1 -> Data Logging Bus1/7  "Thruster_ON_Count"
  Data Store Read146/1 -> Data Logging Bus1/8  "Control_Law_Enabler"
  Data Store Read89/1 -> Data Logging Bus1/9  "RED_Path"
  Data Store Read166/1 -> Data Logging Bus1/10  "ARM_Control_Mode"
  Data Store Read163/1 -> Data Logging Bus1/11  "ARM_Controls"
  Data Store Read162/1 -> Data Logging Bus1/12  "ARM_Measured_States"
  Data Store Read170/1 -> Data Logging Bus1/13  "ARM_Path"
  Data Store Read167/1 -> Data Logging Bus1/14  "ARM_Desired_States"
  Data Store Read165/1 -> Data Logging Bus1/15  "BLACK_Controls"
  Data Store Read171/1 -> Data Logging Bus1/16  "BLACK_Saturated_Controls"
  Data Store Read172/1 -> Data Logging Bus1/17  "BLACK_Measured_States_RAW"
  Data Store Read173/1 -> Data Logging Bus1/18  "BLACK_Desired_States"
  Data Store Read174/1 -> Data Logging Bus1/19  "BLACK_IMU_Measurements"
  Data Store Read175/1 -> Data Logging Bus1/20  "Thruster_ON_Count"
  Data Store Read176/1 -> Data Logging Bus1/21  "Control_Law_Enabler"
  Data Store Read177/1 -> Data Logging Bus1/22  "BLACK_Path"
  Data Store Read155/1 -> Data Logging Bus1/23  "BLUE_Controls"
  Data Store Read156/1 -> Data Logging Bus1/24  "BLUE_Saturated_Controls"
  Data Store Read157/1 -> Data Logging Bus1/25  "BLUE_Measured_States_RAW"
  Data Store Read158/1 -> Data Logging Bus1/26  "BLUE_Desired_States"
  Data Store Read159/1 -> Data Logging Bus1/27  "BLUE_IMU_Measurements"
  Data Store Read160/1 -> Data Logging Bus1/28  "Thruster_ON_Count"
  Data Store Read161/1 -> Data Logging Bus1/29  "Control_Law_Enabler"
  Data Store Read164/1 -> Data Logging Bus1/30
  Data Store Read102/1 -> Data Logging Bus1/31  "Float_State"
  Data Store Read103/1 -> Data Logging Bus1/32  "Platform_Identification"
  Data Store Read104/1 -> Data Logging Bus1/33  "Simulation_Flag"
  Data Store Read124/1 -> Data Logging Bus1/35  "Target_Holding_Radius"
  Data Store Read150/1 -> Data Logging Bus1/39  "Target_Trajectory"
  Data Store Read122/1 -> Data Logging Bus1/36  "Controls"
  Data Store Read123/1 -> Data Logging Bus1/37  "Solver_Result"
  Data Store Read151/1 -> Data Logging Bus1/34  "Docking_Enabler"
  Data Store Read125/1 -> Data Logging Bus1/38  "Optimization_Variable"
  Data Store Read83/1 -> Data Logging Bus1/40  "RED_Estimated_States"
  Data Store Read105/1 -> Reshape17/1
  Reshape17/1 -> Data Logging Bus1/41  "RED_Estimated_Covar"
  Data Store Read120/1 -> Data Logging Bus1/44  "BLUE_Estimated_States"
  Data Store Read126/1 -> Reshape19/1
  Data Store Read135/1 -> Reshape18/1
  Data Store Read136/1 -> Data Logging Bus1/42  "BLACK_Estimated_States"
  Reshape18/1 -> Data Logging Bus1/43  "BLACK_Estimated_Covar"
  Reshape19/1 -> Data Logging Bus1/45  "BLUE_Estimated_Covar"
  Data Store Read82/1 -> Data Logging Bus1/46  "QMEKFx"
  Data Store Read97/1 -> Reshape20/1
  Reshape20/1 -> Data Logging Bus1/47  "QMEKFP"
  Data Store Read130/1 -> Data Logging Bus1/48  "QMEKFt"
  Data Store Read108/1 -> Data Logging Bus1/49  "QMEKFerror"
  Data Store Read119/1 -> Data Logging Bus1/50  "QMEKFNIS"
  Data Store Read128/1 -> Data Logging Bus1/55  "STQMEKFNIS"
  Data Store Read127/1 -> Data Logging Bus1/54  "STQMEKFerror"
  Data Store Read117/1 -> Reshape9/1
  Data Store Read118/1 -> Data Logging Bus1/53  "STQMEKFt"
  Reshape9/1 -> Data Logging Bus1/52  "STQMEKFP"
  Data Store Read85/1 -> Data Logging Bus1/51  "STQMEKFx"
  Reshape12/1 -> Data Logging Bus1/57  "DQMEKFP"
  Data Store Read116/1 -> Data Logging Bus1/56  "DQMEKFx"
  Data Store Read131/1 -> Data Logging Bus1/58  "DQMEKFt"
  Data Store Read114/1 -> Data Logging Bus1/59  "DQMEKFerror"
  Data Store Read115/1 -> Data Logging Bus1/60  "DQMEKFNIS"
  Data Store Read129/1 -> Reshape12/1
  Data Store Read137/1 -> Data Logging Bus1/64  "STDQMEKFerror"
  Data Store Read95/1 -> Reshape11/1
  Data Store Read138/1 -> Data Logging Bus1/65  "STDQMEKFNIS"
  Data Store Read96/1 -> Data Logging Bus1/63  "STDQMEKFt"
  Data Store Read84/1 -> Data Logging Bus1/61  "STDQMEKFx"
  Reshape11/1 -> Data Logging Bus1/62  "STDQMEKFP"
  Data Store Read134/1 -> Reshape21/1  "Error"
  Data Store Read142/1 -> Data Logging Bus1/71  "RMEKFNIS"
  Data Store Read132/1 -> Data Logging Bus1/68  "RMEKFt"
  Data Store Read86/1 -> Data Logging Bus1/70  "RMEKFerror"
  Data Store Read90/1 -> Reshape10/1
  Data Store Read88/1 -> Data Logging Bus1/66  "RMEKFx"
  Data Store Read178/1 -> Data Logging Bus1/74  "STRMEKFt"
  Data Store Read181/1 -> Data Logging Bus1/77  "STRMEKFNIS"
  Data Store Read168/1 -> Reshape22/1
  Data Store Read180/1 -> Data Logging Bus1/76  "STRMEKFerror"
  Data Store Read179/1 -> Reshape23/1
  Reshape22/1 -> Data Logging Bus1/73  "STRMEKFP"
  Reshape23/1 -> Data Logging Bus1/75  "STRMEKFR"
  Data Store Read152/1 -> Data Logging Bus1/72  "STRMEKFx"
  Reshape10/1 -> Data Logging Bus1/67  "RMEKFP"
  Reshape21/1 -> Data Logging Bus1/69  "RMEKFR"
  Data Store Read92/1 -> Data Logging Bus1/82  "Vis_q"
  Data Store Read94/1 -> Data Logging Bus1/78  "Vis_q_zoh"
  Data Store Read93/1 -> Data Logging Bus1/83  "Vis_x"
  Data Store Read98/1 -> Data Logging Bus1/79  "Vis_x_zoh"
  Data Store Read101/1 -> Data Logging Bus1/81  "CNNError"
  Data Store Read100/1 -> Data Logging Bus1/80  "Conf_zoh"
  Data Store Read99/1 -> Data Logging Bus1/84  "Conf"
  Data Logging Bus/1 -> To Workspace1/1, Data Logger1/1
  Subsystem8/1(y) -> Bus Creator1/5  "NIS"
  Subsystem3/1(y) -> Bus Creator2/5  "NIS"
  Subsystem11/1(y) -> Bus Creator5/6  "NIS"
  Subsystem4/1(y) -> Bus Creator6/6  "NIS"
  Subsystem1/1(y) -> Bus Creator3/5  "NIS"
  Subsystem17/1(y) -> Bus Creator4/5  "NIS"
  Subsystem13/1(y) -> CNN_ZOH/3  "Confidence"
  Subsystem14/1(y) -> CNN/3  "Confidence"
  Data Store Read30/1 -> CNN/2  "State"
  Data Store Read29/1 -> CNN/1  "Quat"
  Reshape13/1 -> Bus Creator2/1  "State"
  Reshape14/1 -> Bus Creator3/1  "State"

== system MPC/Debugger1 ==
  Change BLACK Behavior : Subsystem  TreatAsAtomicUnit=on
  Change BLUE Behavior : Subsystem  TreatAsAtomicUnit=on
  Change RED Behavior : Subsystem  TreatAsAtomicUnit=on
  Data Store Read : DataStoreRead  DataStoreName=WhoAmI  IndexOptions=Index vector (dialog)  Indices=1  OutputSizes=1
  Data Store Read1 : DataStoreRead  DataStoreName=isSim  IndexOptions=Index vector (dialog)  Indices=1  OutputSizes=1
  This IF block determines whether or not to run the BLACK sim/exp : If  NumInputs=2  IfExpression=u1 == 2 & u2 == 0  ShowElse=off
  This IF block determines whether or not to run the BLUE sim/exp : If  NumInputs=2  IfExpression=u1 == 3 & u2 == 0  ShowElse=off
  "This IF block determines whether or not to run the RED sim/exp " : If  NumInputs=2  IfExpression=u1 == 1 & u2 == 0  ShowElse=off
  wires:
  Data Store Read1/1 -> This IF block determines whether or not to run the BLACK sim/exp/2, This IF block determines whether or not to run the BLUE sim/exp/2, "This IF block determines whether or not to run the RED sim/exp "/2
  Data Store Read/1 -> This IF block determines whether or not to run the BLUE sim/exp/1, This IF block determines whether or not to run the BLACK sim/exp/1, "This IF block determines whether or not to run the RED sim/exp "/1
  "This IF block determines whether or not to run the RED sim/exp "/1 -> Change RED Behavior/Action
  This IF block determines whether or not to run the BLACK sim/exp/1 -> Change BLACK Behavior/Action
  This IF block determines whether or not to run the BLUE sim/exp/1 -> Change BLUE Behavior/Action

== system MPC/Float Code ==
  note: In this subsection, the "if" statements are used to determine two things: 1) whether or not a simulation is begin performed,
      | then 2) if an experiment is being performed, then which platform is the diagram compiled on. The "IdentifyPlatform" variable
      | is obtained from a text file location on each platform; each text file contains a unique identifier for each platform.
  Data Store Read : DataStoreRead  DataStoreName=isSim  IndexOptions=Index vector (dialog)  Indices=1  OutputSizes=1
  Enable Pucks : Subsystem  TreatAsAtomicUnit=on
  This IF block determines whether or not to run the exp code : If  IfExpression=u1 == 0  ShowElse=off
  wires:
  Data Store Read/1 -> This IF block determines whether or not to run the exp code/1
  This IF block determines whether or not to run the exp code/1 -> Enable Pucks/Action

== system MPC/Gyro.//Accel. Code ==
  Data Store Read1 : DataStoreRead  DataStoreName=isSim  IndexOptions=Index vector (dialog)  Indices=1  OutputSizes=1
  Log Gyro/Accel : Subsystem  TreatAsAtomicUnit=on
  This IF block determines whether or not to run the exp code : If  IfExpression=u1 == 0  ShowElse=off
  wires:
  This IF block determines whether or not to run the exp code/1 -> Log Gyro/Accel/Action
  Data Store Read1/1 -> This IF block determines whether or not to run the exp code/1

== system MPC/Manipulator Encoder Data ==
  note: This if statement checks if a simulation is being performed. If not, it also checks that this code is being run on the RED platform. If it is, then the arm encoders are used to collect the joint angles. NOTE, the encoder data is collected very slowly, about 0.5 Hz. When the diagram is running faster then this collection rate, previous values of the encoder are held constant.
  Change ARM Behavior : Subsystem  TreatAsAtomicUnit=on
  Data Store Read1 : DataStoreRead  DataStoreName=WhoAmI  IndexOptions=Index vector (dialog)  Indices=1  OutputSizes=1
  Data Store Read2 : DataStoreRead  DataStoreName=isSim  IndexOptions=Index vector (dialog)  Indices=1  OutputSizes=1
  "This IF block determines whether or not to run the RED sim/exp " : If  NumInputs=2  IfExpression=u1 == 1 & u2 == 0  ShowElse=off
  wires:
  Data Store Read2/1 -> "This IF block determines whether or not to run the RED sim/exp "/2
  "This IF block determines whether or not to run the RED sim/exp "/1 -> Change ARM Behavior/Action
  Data Store Read1/1 -> "This IF block determines whether or not to run the RED sim/exp "/1

== system MPC/Model Predictive Control ==
  Enable : EnablePort
  Model Predictive Control : Subsystem  TreatAsAtomicUnit=on  SystemSampleTime=T_d

== system MPC/PhaseSpace Camera Code ==
  note: In this subsection, the "if" statement is used to determine if this is a simulation or not. If it is not a simulation, then code is run to receive PhaseSpace camera data via UDP. The PhaseSpace code is currently a standalone executable that should not need to be modified by most users. The code sends all data for all platforms to each platform near simultaneously. If this is a simulation, then no data is required, but a continuous clock is created.
  Data Store Read2 : DataStoreRead  DataStoreName=isSim  IndexOptions=Index vector (dialog)  Indices=1  OutputSizes=1
  "If performing an experiment, grab the PhaseSpace data. Otherwise, use a clock to set time in SIM." : If  IfExpression=u1 == 0  ElseIfExpressions=u1 == 1  ShowElse=off
  Initialize Universal Time (Simulation) : Subsystem  TreatAsAtomicUnit=on
  Use Hardware to Obtain States : Subsystem  TreatAsAtomicUnit=on
  wires:
  Data Store Read2/1 -> "If performing an experiment, grab the PhaseSpace data. Otherwise, use a clock to set time in SIM."/1
  "If performing an experiment, grab the PhaseSpace data. Otherwise, use a clock to set time in SIM."/2 -> Initialize Universal Time (Simulation)/Action
  "If performing an experiment, grab the PhaseSpace data. Otherwise, use a clock to set time in SIM."/1 -> Use Hardware to Obtain States/Action
